simulink model "vfs_matlab"  (R2022a)
settings: Solver=FixedStepAuto  StartTime=0.0  StopTime=tend  FixedStep=0.02  RelTol=1e-3
undefined symbols (not defined in the file): alpha, center1, center2, center3, epsilon1, epsilon2, epsilon3, gd, Kc, psi0, pwo_init, scale1, scale2, scale3, switchingPoints, switchingWidth, T, v1, v2, v3, var_max
libraries: simlib_vpc_basic x23, simlib_vpc_coremath x14, simlib_vpc_gp x7
settings Model: Creator=marco  LastModifiedBy=marco
settings DebuggingCC: AlgebraicLoopMsg=none  ArtificialAlgebraicLoopMsg=none  UnconnectedInputMsg=warning  UnconnectedOutputMsg=warning  UnconnectedLineMsg=warning
settings RTWCC: DLArmComputeVersion=19.05

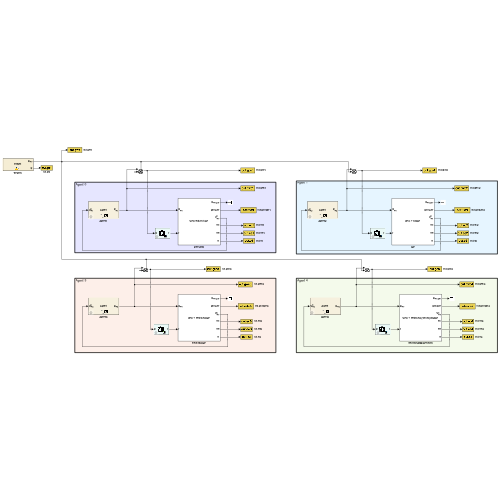
[thumbnail: Simulink's stored preview of the top-level diagram]
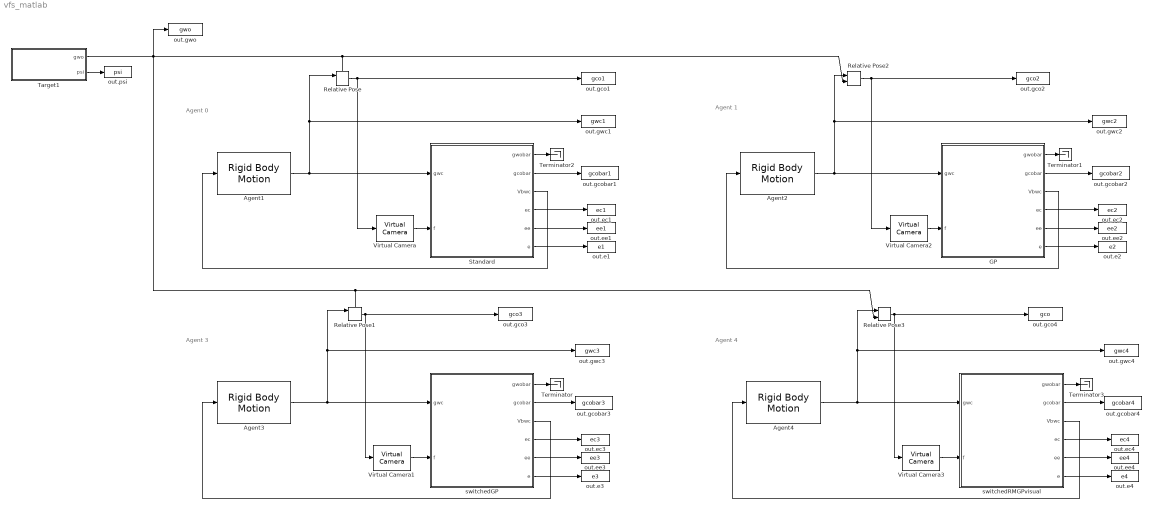
== system vfs_matlab ==
  note: Agent 3
  note: Agent 1
  note: Agent 0
  note: Agent 4
  Agent1 : simlib_vpc_basic/Rigid Body Motion  rbmtype=agent  agentnumber=1  projection=on  show_dg=off  g0=gwc_init
      settings: SourceProductName=VPC Library
  Agent2 : simlib_vpc_basic/Rigid Body Motion  rbmtype=agent  agentnumber=2  projection=on  show_dg=off  g0=gwc_init
      settings: SourceProductName=VPC Library
  Agent3 : simlib_vpc_basic/Rigid Body Motion  rbmtype=agent  agentnumber=3  projection=on  show_dg=off  g0=gwc_init
      settings: SourceProductName=VPC Library
  Agent4 : simlib_vpc_basic/Rigid Body Motion  rbmtype=agent  agentnumber=4  projection=on  show_dg=off  g0=gwc_init
      settings: SourceProductName=VPC Library
  GP : Subsystem
      mask Display:
      | disp('VPC + fullGP','texmode','on')
      | 
      | % Label ports
      | port_label('input',1,'g_{wc}','texmode','on')
      | port_label('input',2,'f','texmode','on')
      | port_label('output',1,'g_{wo,bar}','texmode','on')
      | port_label('output',2,'gco,bar','texmode','on')
      | port_label('output',3,'V^b_{wc}','texmode','on')
      | port_label('output',4,'ec','texmode','on')
      | port_label('output',5,'ee','texmode','on')
      | port_label('output',6,'e','texmode','on')
  Relative Pose{,1..3} (4 alike) : simlib_vpc_coremath/Relative Pose
      settings: SourceProductName=VPC Library
  Standard : Subsystem
      mask Display:
      | disp('VPC without GP','texmode','on')
      | 
      | % Label ports
      | port_label('input',1,'g_{wc}','texmode','on')
      | port_label('input',2,'f','texmode','on')
      | port_label('output',1,'g_{wo,bar}','texmode','on')
      | port_label('output',2,'gco,bar','texmode','on')
      | port_label('output',3,'V^b_{wc}','texmode','on')
      | port_label('output',4,'ec','texmode','on')
      | port_label('output',5,'ee','texmode','on')
      | port_label('output',6,'e','texmode','on')
  Target1 : Subsystem
      mask Display:
      | % Glitch in Matlab: If you define a line whose starting point and end point
      | % is equal, then the entire mask block is plotted in bold
      | plot([0,0],[0,0])
      | 
      | % Draw Box
      | plot([0,1,1,0,0],[0,0,1,1,0])
      | 
      | % Write label
      | disp('Target','texmode','on')
      | 
      | % Image
      | p=get_param(gcb,'Position');
      | size = min(p(3:4)-p(1:2));
      | blkscale = abs((p(3)-p(1)) / (p(4)-p(2)));
      | if abs((p(3)-p(1))) > abs((p(4)-p(2))) % block is horizontal
      |     scale = .5*[1/blkscale .6];
      | else % block is vertical
      |     scale = .5*[1 .6*blkscale];
      | end
      | pos = [1-scale(1) 0.1]/2;
      | image('ico_target.png',[pos scale],'off')
      | 
      | % Label ports
      | port_label('output',1,'g_{wo}','texmode','on')
      | port_label('output',2,'\psi','texmode','on')
  Terminator{,1..3} (4 alike) : Terminator
  Virtual Camera{,1..3} (4 alike) : simlib_vpc_basic/Virtual Camera  camtype=Pinhole  po=fp  lambda=lambda
      settings: SourceProductName=VPC Library
  out.e1 : ToWorkspace  VariableName=e1  SaveFormat=Structure With Time  SampleTime=-1
  out.e2 : ToWorkspace  VariableName=e2  SaveFormat=Structure With Time  SampleTime=-1
  out.e3 : ToWorkspace  VariableName=e3  SaveFormat=Structure With Time  SampleTime=-1
  out.e4 : ToWorkspace  VariableName=e4  SaveFormat=Structure With Time  SampleTime=-1
  out.ec1 : ToWorkspace  VariableName=ec1  SaveFormat=Structure With Time  SampleTime=-1
  out.ec2 : ToWorkspace  VariableName=ec2  SaveFormat=Structure With Time  SampleTime=-1
  out.ec3 : ToWorkspace  VariableName=ec3  SaveFormat=Structure With Time  SampleTime=-1
  out.ec4 : ToWorkspace  VariableName=ec4  SaveFormat=Structure With Time  SampleTime=-1
  out.ee1 : ToWorkspace  VariableName=ee1  SaveFormat=Structure With Time  SampleTime=-1
  out.ee2 : ToWorkspace  VariableName=ee2  SaveFormat=Structure With Time  SampleTime=-1
  out.ee3 : ToWorkspace  VariableName=ee3  SaveFormat=Structure With Time  SampleTime=-1
  out.ee4 : ToWorkspace  VariableName=ee4  SaveFormat=Structure With Time  SampleTime=-1
  out.gco1 : ToWorkspace  VariableName=gco1  SaveFormat=Structure With Time  SampleTime=-1
  out.gco2 : ToWorkspace  VariableName=gco2  SaveFormat=Structure With Time  SampleTime=-1
  out.gco3 : ToWorkspace  VariableName=gco3  SaveFormat=Structure With Time  SampleTime=-1
  out.gco4 : ToWorkspace  VariableName=gco  SaveFormat=Structure With Time  SampleTime=-1
  out.gcobar1 : ToWorkspace  VariableName=gcobar1  SaveFormat=Structure With Time  SampleTime=-1
  out.gcobar2 : ToWorkspace  VariableName=gcobar2  SaveFormat=Structure With Time  SampleTime=-1
  out.gcobar3 : ToWorkspace  VariableName=gcobar3  SaveFormat=Structure With Time  SampleTime=-1
  out.gcobar4 : ToWorkspace  VariableName=gcobar4  SaveFormat=Structure With Time  SampleTime=-1
  out.gwc1 : ToWorkspace  VariableName=gwc1  SaveFormat=Structure With Time  SampleTime=-1
  out.gwc2 : ToWorkspace  VariableName=gwc2  SaveFormat=Structure With Time  SampleTime=-1
  out.gwc3 : ToWorkspace  VariableName=gwc3  SaveFormat=Structure With Time  SampleTime=-1
  out.gwc4 : ToWorkspace  VariableName=gwc4  SaveFormat=Structure With Time  SampleTime=-1
  out.gwo : ToWorkspace  VariableName=gwo  SaveFormat=Structure With Time  SampleTime=-1
  out.psi : ToWorkspace  VariableName=psi  SaveFormat=Structure With Time  SampleTime=-1
  switchedGP : Subsystem
      mask Display:
      | disp('VPC + switchedGP','texmode','on')
      | 
      | % Label ports
      | port_label('input',1,'g_{wc}','texmode','on')
      | port_label('input',2,'f','texmode','on')
      | port_label('output',1,'g_{wo,bar}','texmode','on')
      | port_label('output',2,'gco,bar','texmode','on')
      | port_label('output',3,'V^b_{wc}','texmode','on')
      | port_label('output',4,'ec','texmode','on')
      | port_label('output',5,'ee','texmode','on')
      | port_label('output',6,'e','texmode','on')
  switchedRMGPvisual : Subsystem
      mask Display:
      | disp('VPC + switched (visual) RMGP','texmode','on')
      | 
      | % Label ports
      | port_label('input',1,'g_{wc}','texmode','on')
      | port_label('input',2,'f','texmode','on')
      | port_label('output',1,'g_{wo,bar}','texmode','on')
      | port_label('output',2,'gco,bar','texmode','on')
      | port_label('output',3,'V^b_{wc}','texmode','on')
      | port_label('output',4,'ec','texmode','on')
      | port_label('output',5,'ee','texmode','on')
      | port_label('output',6,'e','texmode','on')
  wires:
  Relative Pose2/1 -> Virtual Camera2/1, out.gco2/1
  Relative Pose/1 -> Virtual Camera/1, out.gco1/1
  GP/2(gcobar) -> out.gcobar2/1
  switchedGP/4(ec) -> out.ec3/1
  Relative Pose1/1 -> out.gco3/1, Virtual Camera1/1
  Agent3/1 -> switchedGP/1(gwc), out.gwc3/1, Relative Pose1/1
  Virtual Camera/1 -> Standard/2(f)
  switchedGP/2(gcobar) -> out.gcobar3/1
  Virtual Camera2/1 -> GP/2(f)
  switchedGP/5(ee) -> out.ee3/1
  GP/4(ec) -> out.ec2/1
  switchedGP/6(e) -> out.e3/1
  Virtual Camera1/1 -> switchedGP/2(f)
  Agent1/1 -> Standard/1(gwc), out.gwc1/1, Relative Pose/1
  Standard/6(e) -> out.e1/1
  Target1/1(gwo) -> Relative Pose2/2, Relative Pose/2, out.gwo/1, Relative Pose3/2, Relative Pose1/2
  Standard/4(ec) -> out.ec1/1
  Standard/5(ee) -> out.ee1/1
  Agent2/1 -> GP/1(gwc), out.gwc2/1, Relative Pose2/1
  Standard/2(gcobar) -> out.gcobar1/1
  GP/5(ee) -> out.ee2/1
  GP/6(e) -> out.e2/1
  Standard/3(Vbwc) -> Agent1/1
  switchedGP/3(Vbwc) -> Agent3/1
  GP/3(Vbwc) -> Agent2/1
  switchedGP/1(gwobar) -> Terminator/1
  GP/1(gwobar) -> Terminator1/1
  Standard/1(gwobar) -> Terminator2/1
  switchedRMGPvisual/4(ec) -> out.ec4/1
  switchedRMGPvisual/6(e) -> out.e4/1
  switchedRMGPvisual/5(ee) -> out.ee4/1
  Relative Pose3/1 -> out.gco4/1, Virtual Camera3/1
  switchedRMGPvisual/2(gcobar) -> out.gcobar4/1
  Agent4/1 -> switchedRMGPvisual/1(gwc), out.gwc4/1, Relative Pose3/1
  switchedRMGPvisual/3(Vbwc) -> Agent4/1
  Virtual Camera3/1 -> switchedRMGPvisual/2(f)
  switchedRMGPvisual/1(gwobar) -> Terminator3/1
  Target1/2(psi) -> out.psi/1

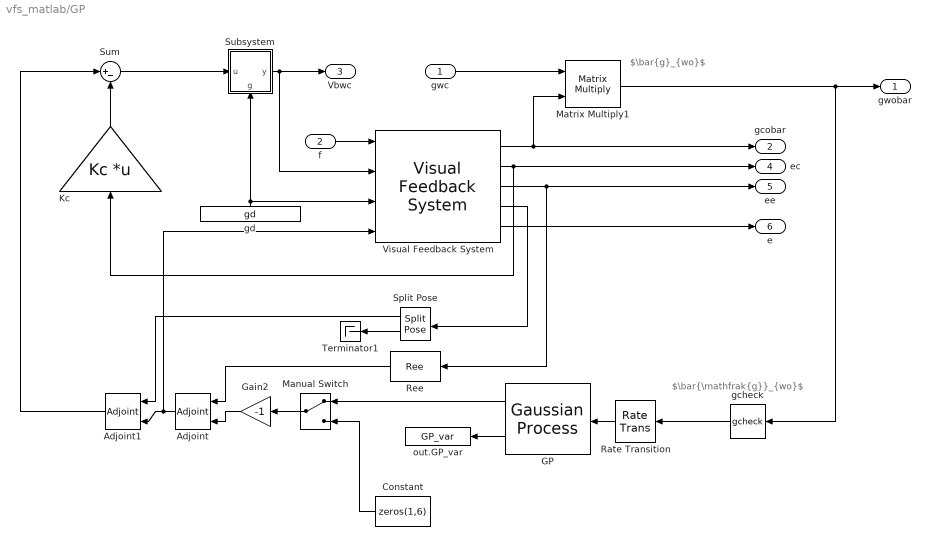
== system vfs_matlab/GP ==
  note: $\bar{g}_{wo}$
  note: $\bar{\mathfrak{g}}_{wo}$
  gwc : Inport
  f : Inport  Port=2
  Adjoint : simlib_vpc_basic/Adjoint  adjointtype=orientation
      settings: SourceProductName=VPC Library
  Adjoint1 : simlib_vpc_basic/Adjoint  adjointtype=orientation
      settings: SourceProductName=VPC Library
  Constant : Constant  Value=zeros(1,6)
  GP : simlib_vpc_gp/Gaussian Process  X=X_GP  Y=Y_GP  sn=sn_GP  kernel=Squared Exponential ARD  hyp=hyp_GP  show_mean=on  show_variance=on  inv_fallback=off
      settings: SourceProductName=VPC Library
  Gain2 : Gain  Gain=-1
  Kc : Gain  Gain=Kc  Multiplication=Matrix(K*u) (u vector)
  Manual Switch : ManualSwitch
  Matrix Multiply1 : Product  Multiplication=Matrix(*)
  Rate Transition : RateTransition
  Ree : simlib_vpc_coremath/Ree
      settings: SourceProductName=VPC Library
  Split Pose : simlib_vpc_coremath/Split Pose  show_R=on  show_p=on
      settings: SourceProductName=VPC Library
  Subsystem : Subsystem
      settings: PortSchema="{\"entries\":[{\"content\":{\"sides\":[{\"content\":{\"connectorIds\":[\"In1\"]},\"type\":\"ConnectorPlacement.EquallySpacedRectSide\",\"uuid\":\"72e68008-5c4a-43a9-a560-64c6a31a0c08\"},{\"content\":{\"connectorIds\":[\"Out1\"],\"side\":\"RIGHT\"},\"type\":\"ConnectorPlacement.EquallySpacedRectSide\",\"uuid\":\"da07f5ff-2b2c-4c55-a2f2-34e133777503\"},{\"content\":{\"connectorIds\":[],\"side\":\"TOP\"},\"type\":\"ConnectorPlacement.EquallySpacedRectSide\",\"uuid\":\"6d174428-4364-4e89-aba7-4e9864808ab5\"},{\"content\":{\"connectorIds\":[\"In2\"],\"side\":\"BOTTOM\"},\"type\":\"ConnectorPlacement.EquallySpacedRectSide\",\"uuid\":\"f9633104-9c11-4d21-90a7-e0f886d9e92d\"},{\"content\":{\"connectorIds\":[],\"side\":\"HIDDEN\"},\"type\":\"ConnectorPlacement.EquallySpacedRectSide\",\"uuid\":\"662f08ae-9279-4a4f-85ea-81d97ead27d9\"}]},\"type\":\"ConnectorPlacement.EquallySpacedConnector\",\"uuid\":\"f3cd156c-cccd-47c6-b81c-6113f78efd58\"}],\"packageUris\":[\"http://schema.mathworks.com/mf0/Connector/R2020b\"],\"version\":\"1.0\"}"
      mask Display:
      | % Glitch in Matlab: If you define a line whose starting point and end point
      | % is equal, then the entire mask block is plotted in bold
      | plot([0,0],[0,0])
      | 
      | % Draw box
      | indent = 0.3;
      | ang=[0:0.2:pi/2, pi/2];
      | plot([0,1-indent],[0,0])
      | xp=indent*sin(ang)+1-indent;
      | yp=indent-indent*cos(ang);
      | plot(xp,yp);
      | plot([1,1,indent],[indent,1,1])
      | xp=indent-indent*sin(ang);
      | yp=1-indent+indent*cos(ang);
      | plot(xp,yp);
      | plot([0,0],[1-indent,0])
      | 
      | % Write label & ports
      | disp('-Ad_{(g_d)}','texmode','on')
      | text(0.5,0.2,'\fontsize{7}g_d','texmode','on')
  Sum : Sum  Inputs=|+-
  Terminator1 : Terminator
  Visual Feedback System : simlib_vpc_basic/Visual Feedback System  gd_source=external  gd_value=[eye(4,3),ones(4,1)]  gcobar0=gco_init  Ke_source=internal  Ke=Ke  projection=on  camtype=Pinhole  fo=fp  lambda=lambda  show_Vbwo=off  show_ec=on  show_gce=on  show_ee=on  show_gee=off  show_e=on  show_nu=off  show_dgcobar=off  show_ue_aux=on
      settings: SourceProductName=VPC Library
  gcheck : simlib_vpc_coremath/gcheck
      settings: SourceProductName=VPC Library
  gd : Constant  Value=gd
  out.GP_var : ToWorkspace  VariableName=GP_var  SaveFormat=Structure With Time  SampleTime=-1
  gwobar : Outport
  gcobar : Outport  Port=2
  Vbwc : Outport  Port=3
  ec : Outport  Port=4
  ee : Outport  Port=5
  e : Outport  Port=6
  wires:
  f/1 -> Visual Feedback System/1
  Matrix Multiply1/1 -> gcheck/1, gwobar/1
  Subsystem/1(y) -> Vbwc/1, Visual Feedback System/2
  gwc/1 -> Matrix Multiply1/1
  Visual Feedback System/5 -> e/1
  Kc/1 -> Sum/2
  Visual Feedback System/2 -> ec/1, Kc/1
  Visual Feedback System/3 -> Ree/1, ee/1
  gd/1 -> Subsystem/2(g), Visual Feedback System/3
  Visual Feedback System/1 -> Matrix Multiply1/2, gcobar/1
  Split Pose/1 -> Adjoint1/2
  Rate Transition/1 -> GP/1
  Adjoint/1 -> Visual Feedback System/4, Adjoint1/1
  Ree/1 -> Adjoint/2
  Split Pose/2 -> Terminator1/1
  Gain2/1 -> Adjoint/1
  Manual Switch/1 -> Gain2/1
  Sum/1 -> Subsystem/1(u)
  Adjoint1/1 -> Sum/1
  Visual Feedback System/4 -> Split Pose/1
  GP/2 -> out.GP_var/1
  gcheck/1 -> Rate Transition/1
  GP/1 -> Manual Switch/1
  Constant/1 -> Manual Switch/2

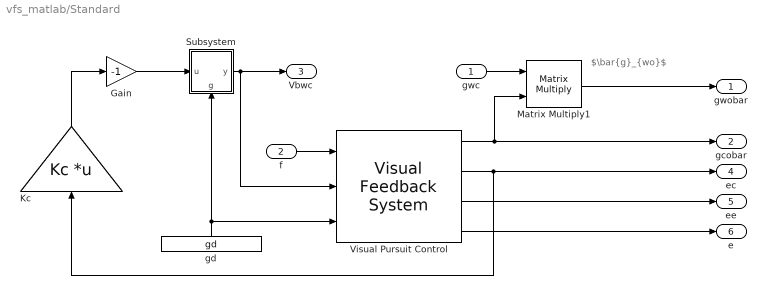
== system vfs_matlab/Standard ==
  note: $\bar{g}_{wo}$
  gwc : Inport
  f : Inport  Port=2
  Gain : Gain  Gain=-1
  Kc : Gain  Gain=Kc  Multiplication=Matrix(K*u) (u vector)
  Matrix Multiply1 : Product  Multiplication=Matrix(*)
  Subsystem : Subsystem
      settings: PortSchema="{\"entries\":[{\"content\":{\"sides\":[{\"content\":{\"connectorIds\":[\"In1\"]},\"type\":\"ConnectorPlacement.EquallySpacedRectSide\",\"uuid\":\"72e68008-5c4a-43a9-a560-64c6a31a0c08\"},{\"content\":{\"connectorIds\":[\"Out1\"],\"side\":\"RIGHT\"},\"type\":\"ConnectorPlacement.EquallySpacedRectSide\",\"uuid\":\"da07f5ff-2b2c-4c55-a2f2-34e133777503\"},{\"content\":{\"connectorIds\":[],\"side\":\"TOP\"},\"type\":\"ConnectorPlacement.EquallySpacedRectSide\",\"uuid\":\"6d174428-4364-4e89-aba7-4e9864808ab5\"},{\"content\":{\"connectorIds\":[\"In2\"],\"side\":\"BOTTOM\"},\"type\":\"ConnectorPlacement.EquallySpacedRectSide\",\"uuid\":\"f9633104-9c11-4d21-90a7-e0f886d9e92d\"},{\"content\":{\"connectorIds\":[],\"side\":\"HIDDEN\"},\"type\":\"ConnectorPlacement.EquallySpacedRectSide\",\"uuid\":\"662f08ae-9279-4a4f-85ea-81d97ead27d9\"}]},\"type\":\"ConnectorPlacement.EquallySpacedConnector\",\"uuid\":\"f3cd156c-cccd-47c6-b81c-6113f78efd58\"}],\"packageUris\":[\"http://schema.mathworks.com/mf0/Connector/R2020b\"],\"version\":\"1.0\"}"
      mask Display:
      | % Glitch in Matlab: If you define a line whose starting point and end point
      | % is equal, then the entire mask block is plotted in bold
      | plot([0,0],[0,0])
      | 
      | % Draw box
      | indent = 0.3;
      | ang=[0:0.2:pi/2, pi/2];
      | plot([0,1-indent],[0,0])
      | xp=indent*sin(ang)+1-indent;
      | yp=indent-indent*cos(ang);
      | plot(xp,yp);
      | plot([1,1,indent],[indent,1,1])
      | xp=indent-indent*sin(ang);
      | yp=1-indent+indent*cos(ang);
      | plot(xp,yp);
      | plot([0,0],[1-indent,0])
      | 
      | % Write label & ports
      | disp('-Ad_{(g_d)}','texmode','on')
      | text(0.5,0.2,'\fontsize{7}g_d','texmode','on')
  Visual Pursuit Control : simlib_vpc_basic/Visual Feedback System  gd_source=external  gd_value=[eye(4,3),ones(4,1)]  gcobar0=gco_init  Ke_source=internal  Ke=Ke  projection=on  camtype=Pinhole  fo=fp  lambda=lambda  show_Vbwo=off  show_ec=on  show_gce=off  show_ee=on  show_gee=off  show_e=on  show_nu=off  show_dgcobar=off  show_ue_aux=off
      settings: SourceProductName=VPC Library
  gd : Constant  Value=gd
  gwobar : Outport
  gcobar : Outport  Port=2
  Vbwc : Outport  Port=3
  ec : Outport  Port=4
  ee : Outport  Port=5
  e : Outport  Port=6
  wires:
  f/1 -> Visual Pursuit Control/1
  Matrix Multiply1/1 -> gwobar/1
  Subsystem/1(y) -> Vbwc/1, Visual Pursuit Control/2
  gwc/1 -> Matrix Multiply1/1
  Kc/1 -> Gain/1
  Visual Pursuit Control/4 -> e/1
  Gain/1 -> Subsystem/1(u)
  Visual Pursuit Control/2 -> ec/1, Kc/1
  Visual Pursuit Control/3 -> ee/1
  gd/1 -> Subsystem/2(g), Visual Pursuit Control/3
  Visual Pursuit Control/1 -> gcobar/1, Matrix Multiply1/2

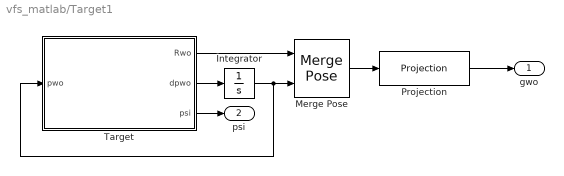
== system vfs_matlab/Target1 ==
  Integrator : Integrator  InitialCondition=pwo_init  ContinuousStateAttributes='pose'
  Merge Pose : simlib_vpc_coremath/Merge Pose
      settings: SourceProductName=VPC Library
  Projection : simlib_vpc_basic/Projection  projectiontype=averaging  inputtype=pose
      settings: SourceProductName=VPC Library
  Target : MATLAB Function  TreatAsAtomicUnit=on  SystemSampleTime=0.02
  gwo : Outport
  psi : Outport  Port=2
  wires:
  Target/1(Rwo) -> Merge Pose/1
  Target/2(dpwo) -> Integrator/1
  Integrator/1 -> Merge Pose/2, Target/1(pwo)
  Projection/1 -> gwo/1
  Merge Pose/1 -> Projection/1
  Target/3(psi) -> psi/1

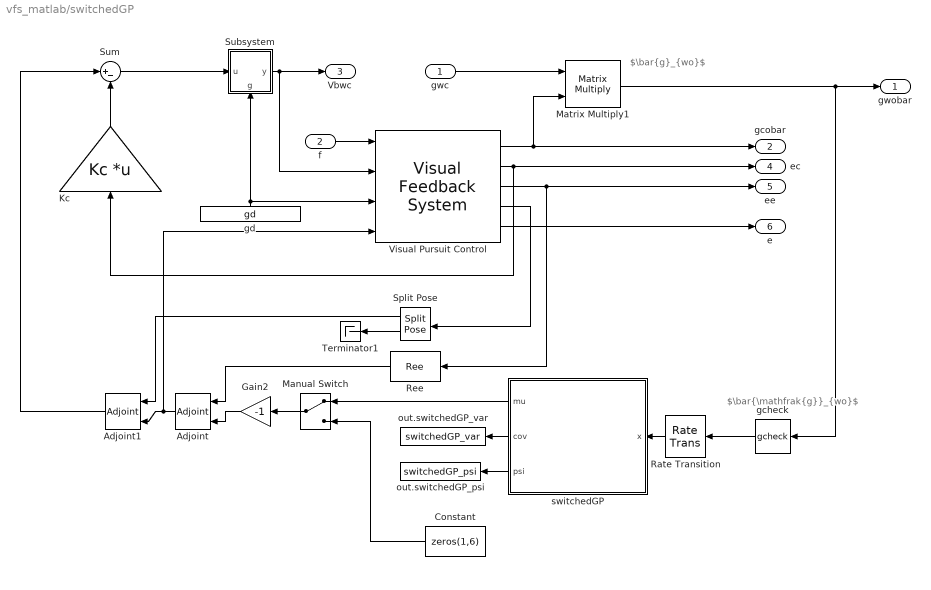
== system vfs_matlab/switchedGP ==
  note: $\bar{g}_{wo}$
  note: $\bar{\mathfrak{g}}_{wo}$
  gwc : Inport
  f : Inport  Port=2
  Adjoint : simlib_vpc_basic/Adjoint  adjointtype=orientation
      settings: SourceProductName=VPC Library
  Adjoint1 : simlib_vpc_basic/Adjoint  adjointtype=orientation
      settings: SourceProductName=VPC Library
  Constant : Constant  Value=zeros(1,6)
  Gain2 : Gain  Gain=-1
  Kc : Gain  Gain=Kc  Multiplication=Matrix(K*u) (u vector)
  Manual Switch : ManualSwitch
  Matrix Multiply1 : Product  Multiplication=Matrix(*)
  Rate Transition : RateTransition
  Ree : simlib_vpc_coremath/Ree
      settings: SourceProductName=VPC Library
  Split Pose : simlib_vpc_coremath/Split Pose  show_R=on  show_p=on
      settings: SourceProductName=VPC Library
  Subsystem : Subsystem
      settings: PortSchema="{\"entries\":[{\"content\":{\"sides\":[{\"content\":{\"connectorIds\":[\"In1\"]},\"type\":\"ConnectorPlacement.EquallySpacedRectSide\",\"uuid\":\"72e68008-5c4a-43a9-a560-64c6a31a0c08\"},{\"content\":{\"connectorIds\":[\"Out1\"],\"side\":\"RIGHT\"},\"type\":\"ConnectorPlacement.EquallySpacedRectSide\",\"uuid\":\"da07f5ff-2b2c-4c55-a2f2-34e133777503\"},{\"content\":{\"connectorIds\":[],\"side\":\"TOP\"},\"type\":\"ConnectorPlacement.EquallySpacedRectSide\",\"uuid\":\"6d174428-4364-4e89-aba7-4e9864808ab5\"},{\"content\":{\"connectorIds\":[\"In2\"],\"side\":\"BOTTOM\"},\"type\":\"ConnectorPlacement.EquallySpacedRectSide\",\"uuid\":\"f9633104-9c11-4d21-90a7-e0f886d9e92d\"},{\"content\":{\"connectorIds\":[],\"side\":\"HIDDEN\"},\"type\":\"ConnectorPlacement.EquallySpacedRectSide\",\"uuid\":\"662f08ae-9279-4a4f-85ea-81d97ead27d9\"}]},\"type\":\"ConnectorPlacement.EquallySpacedConnector\",\"uuid\":\"f3cd156c-cccd-47c6-b81c-6113f78efd58\"}],\"packageUris\":[\"http://schema.mathworks.com/mf0/Connector/R2020b\"],\"version\":\"1.0\"}"
      mask Display:
      | % Glitch in Matlab: If you define a line whose starting point and end point
      | % is equal, then the entire mask block is plotted in bold
      | plot([0,0],[0,0])
      | 
      | % Draw box
      | indent = 0.3;
      | ang=[0:0.2:pi/2, pi/2];
      | plot([0,1-indent],[0,0])
      | xp=indent*sin(ang)+1-indent;
      | yp=indent-indent*cos(ang);
      | plot(xp,yp);
      | plot([1,1,indent],[indent,1,1])
      | xp=indent-indent*sin(ang);
      | yp=1-indent+indent*cos(ang);
      | plot(xp,yp);
      | plot([0,0],[1-indent,0])
      | 
      | % Write label & ports
      | disp('-Ad_{(g_d)}','texmode','on')
      | text(0.5,0.2,'\fontsize{7}g_d','texmode','on')
  Sum : Sum  Inputs=|+-
  Terminator1 : Terminator
  Visual Pursuit Control : simlib_vpc_basic/Visual Feedback System  gd_source=external  gd_value=[eye(4,3),ones(4,1)]  gcobar0=gco_init  Ke_source=internal  Ke=Ke  projection=on  camtype=Pinhole  fo=fp  lambda=lambda  show_Vbwo=off  show_ec=on  show_gce=on  show_ee=on  show_gee=off  show_e=on  show_nu=off  show_dgcobar=off  show_ue_aux=on
      settings: SourceProductName=VPC Library
  gcheck : simlib_vpc_coremath/gcheck
      settings: SourceProductName=VPC Library
  gd : Constant  Value=gd
  out.switchedGP_psi : ToWorkspace  VariableName=switchedGP_psi  SaveFormat=Structure With Time  SampleTime=-1
  out.switchedGP_var : ToWorkspace  VariableName=switchedGP_var  SaveFormat=Structure With Time  SampleTime=-1
  switchedGP : Subsystem
      mask Display:
      | disp('Switched GP','texmode','on')
      | 
      | % Label ports
      | port_label('input',1,'x*','texmode','on')
      | port_label('output',1,'\mu','texmode','on')
      | port_label('output',2,'\Sigma','texmode','on')
      | port_label('output',3,'\psi_{est}','texmode','on')
  gwobar : Outport
  gcobar : Outport  Port=2
  Vbwc : Outport  Port=3
  ec : Outport  Port=4
  ee : Outport  Port=5
  e : Outport  Port=6
  wires:
  f/1 -> Visual Pursuit Control/1
  Matrix Multiply1/1 -> gcheck/1, gwobar/1
  Subsystem/1(y) -> Vbwc/1, Visual Pursuit Control/2
  gwc/1 -> Matrix Multiply1/1
  Visual Pursuit Control/5 -> e/1
  Kc/1 -> Sum/2
  Visual Pursuit Control/2 -> ec/1, Kc/1
  Visual Pursuit Control/3 -> Ree/1, ee/1
  gd/1 -> Subsystem/2(g), Visual Pursuit Control/3
  Visual Pursuit Control/1 -> Matrix Multiply1/2, gcobar/1
  Split Pose/1 -> Adjoint1/2
  Adjoint/1 -> Visual Pursuit Control/4, Adjoint1/1
  Ree/1 -> Adjoint/2
  Split Pose/2 -> Terminator1/1
  Gain2/1 -> Adjoint/1
  Sum/1 -> Subsystem/1(u)
  Adjoint1/1 -> Sum/1
  Visual Pursuit Control/4 -> Split Pose/1
  gcheck/1 -> Rate Transition/1
  switchedGP/3(psi) -> out.switchedGP_psi/1
  Rate Transition/1 -> switchedGP/1(x)
  switchedGP/2(cov) -> out.switchedGP_var/1
  switchedGP/1(mu) -> Manual Switch/1
  Manual Switch/1 -> Gain2/1
  Constant/1 -> Manual Switch/2

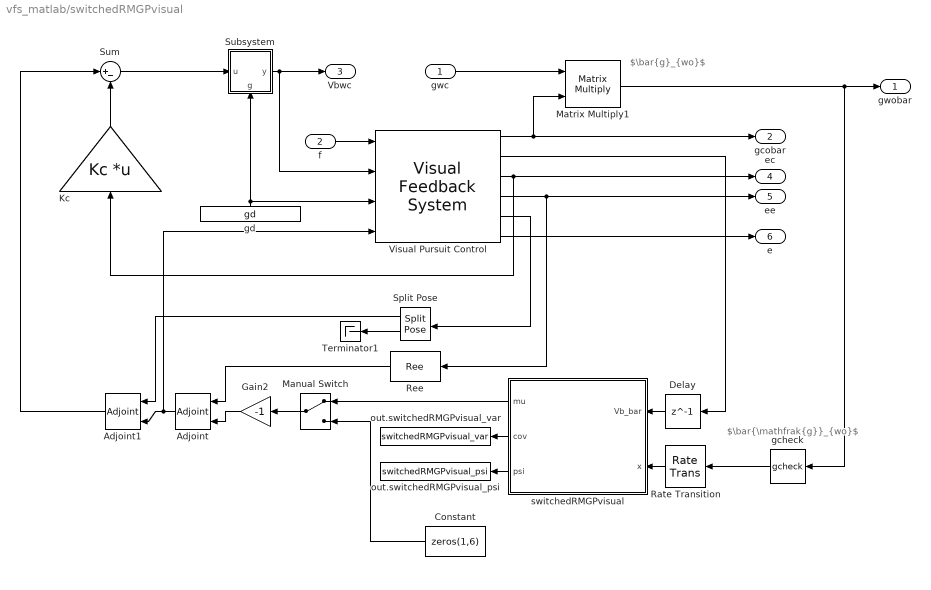
== system vfs_matlab/switchedRMGPvisual ==
  note: $\bar{g}_{wo}$
  note: $\bar{\mathfrak{g}}_{wo}$
  gwc : Inport
  f : Inport  Port=2
  Adjoint : simlib_vpc_basic/Adjoint  adjointtype=orientation
      settings: SourceProductName=VPC Library
  Adjoint1 : simlib_vpc_basic/Adjoint  adjointtype=orientation
      settings: SourceProductName=VPC Library
  Constant : Constant  Value=zeros(1,6)
  Delay : Delay  DelayLength=1
  Gain2 : Gain  Gain=-1
  Kc : Gain  Gain=Kc  Multiplication=Matrix(K*u) (u vector)
  Manual Switch : ManualSwitch
  Matrix Multiply1 : Product  Multiplication=Matrix(*)
  Rate Transition : RateTransition
  Ree : simlib_vpc_coremath/Ree
      settings: SourceProductName=VPC Library
  Split Pose : simlib_vpc_coremath/Split Pose  show_R=on  show_p=on
      settings: SourceProductName=VPC Library
  Subsystem : Subsystem
      settings: PortSchema="{\"entries\":[{\"content\":{\"sides\":[{\"content\":{\"connectorIds\":[\"In1\"]},\"type\":\"ConnectorPlacement.EquallySpacedRectSide\",\"uuid\":\"72e68008-5c4a-43a9-a560-64c6a31a0c08\"},{\"content\":{\"connectorIds\":[\"Out1\"],\"side\":\"RIGHT\"},\"type\":\"ConnectorPlacement.EquallySpacedRectSide\",\"uuid\":\"da07f5ff-2b2c-4c55-a2f2-34e133777503\"},{\"content\":{\"connectorIds\":[],\"side\":\"TOP\"},\"type\":\"ConnectorPlacement.EquallySpacedRectSide\",\"uuid\":\"6d174428-4364-4e89-aba7-4e9864808ab5\"},{\"content\":{\"connectorIds\":[\"In2\"],\"side\":\"BOTTOM\"},\"type\":\"ConnectorPlacement.EquallySpacedRectSide\",\"uuid\":\"f9633104-9c11-4d21-90a7-e0f886d9e92d\"},{\"content\":{\"connectorIds\":[],\"side\":\"HIDDEN\"},\"type\":\"ConnectorPlacement.EquallySpacedRectSide\",\"uuid\":\"662f08ae-9279-4a4f-85ea-81d97ead27d9\"}]},\"type\":\"ConnectorPlacement.EquallySpacedConnector\",\"uuid\":\"f3cd156c-cccd-47c6-b81c-6113f78efd58\"}],\"packageUris\":[\"http://schema.mathworks.com/mf0/Connector/R2020b\"],\"version\":\"1.0\"}"
      mask Display:
      | % Glitch in Matlab: If you define a line whose starting point and end point
      | % is equal, then the entire mask block is plotted in bold
      | plot([0,0],[0,0])
      | 
      | % Draw box
      | indent = 0.3;
      | ang=[0:0.2:pi/2, pi/2];
      | plot([0,1-indent],[0,0])
      | xp=indent*sin(ang)+1-indent;
      | yp=indent-indent*cos(ang);
      | plot(xp,yp);
      | plot([1,1,indent],[indent,1,1])
      | xp=indent-indent*sin(ang);
      | yp=1-indent+indent*cos(ang);
      | plot(xp,yp);
      | plot([0,0],[1-indent,0])
      | 
      | % Write label & ports
      | disp('-Ad_{(g_d)}','texmode','on')
      | text(0.5,0.2,'\fontsize{7}g_d','texmode','on')
  Sum : Sum  Inputs=|+-
  Terminator1 : Terminator
  Visual Pursuit Control : simlib_vpc_basic/Visual Feedback System  gd_source=external  gd_value=[eye(4,3),ones(4,1)]  gcobar0=gco_init  Ke_source=internal  Ke=Ke  projection=on  camtype=Pinhole  fo=fp  lambda=lambda  show_Vbwo=on  show_ec=on  show_gce=on  show_ee=on  show_gee=off  show_e=on  show_nu=off  show_dgcobar=off  show_ue_aux=on
      settings: SourceProductName=VPC Library
  gcheck : simlib_vpc_coremath/gcheck
      settings: SourceProductName=VPC Library
  gd : Constant  Value=gd
  out.switchedRMGPvisual_psi : ToWorkspace  VariableName=switchedRMGPvisual_psi  SaveFormat=Structure With Time  SampleTime=-1
  out.switchedRMGPvisual_var : ToWorkspace  VariableName=switchedRMGPvisual_var  SaveFormat=Structure With Time  SampleTime=-1
  switchedRMGPvisual : Subsystem
      mask Display:
      | disp('Switched GP','texmode','on')
      | 
      | % Label ports
      | port_label('input',1,'V^b_{est}','texmode','on')
      | port_label('input',2,'x*','texmode','on')
      | port_label('output',1,'\mu','texmode','on')
      | port_label('output',2,'\Sigma','texmode','on')
      | port_label('output',3,'\psi_{est}','texmode','on')
  gwobar : Outport
  gcobar : Outport  Port=2
  Vbwc : Outport  Port=3
  ec : Outport  Port=4
  ee : Outport  Port=5
  e : Outport  Port=6
  wires:
  f/1 -> Visual Pursuit Control/1
  Matrix Multiply1/1 -> gwobar/1, gcheck/1
  Subsystem/1(y) -> Vbwc/1, Visual Pursuit Control/2
  gwc/1 -> Matrix Multiply1/1
  Visual Pursuit Control/5 -> Split Pose/1
  Kc/1 -> Sum/2
  Visual Pursuit Control/3 -> ec/1, Kc/1
  Visual Pursuit Control/4 -> Ree/1, ee/1
  gd/1 -> Subsystem/2(g), Visual Pursuit Control/3
  Visual Pursuit Control/1 -> Matrix Multiply1/2, gcobar/1
  Split Pose/1 -> Adjoint1/2
  Adjoint/1 -> Visual Pursuit Control/4, Adjoint1/1
  Ree/1 -> Adjoint/2
  Split Pose/2 -> Terminator1/1
  Gain2/1 -> Adjoint/1
  Sum/1 -> Subsystem/1(u)
  Adjoint1/1 -> Sum/1
  Visual Pursuit Control/6 -> e/1
  gcheck/1 -> Rate Transition/1
  switchedRMGPvisual/3(psi) -> out.switchedRMGPvisual_psi/1
  Rate Transition/1 -> switchedRMGPvisual/2(x)
  switchedRMGPvisual/2(cov) -> out.switchedRMGPvisual_var/1
  switchedRMGPvisual/1(mu) -> Manual Switch/1
  Manual Switch/1 -> Gain2/1
  Constant/1 -> Manual Switch/2
  Delay/1 -> switchedRMGPvisual/1(Vb_bar)
  Visual Pursuit Control/2 -> Delay/1

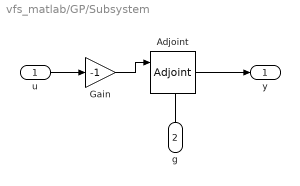
== system vfs_matlab/GP/Subsystem ==
  u : Inport
  g : Inport  Port=2
  Adjoint : simlib_vpc_basic/Adjoint  adjointtype=pose
      settings: SourceProductName=VPC Library
  Gain : Gain  Gain=-1
  y : Outport
  wires:
  Adjoint/1 -> y/1
  u/1 -> Gain/1
  g/1 -> Adjoint/2
  Gain/1 -> Adjoint/1

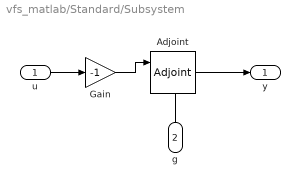
== system vfs_matlab/Standard/Subsystem ==
  u : Inport
  g : Inport  Port=2
  Adjoint : simlib_vpc_basic/Adjoint  adjointtype=pose
      settings: SourceProductName=VPC Library
  Gain : Gain  Gain=-1
  y : Outport
  wires:
  Adjoint/1 -> y/1
  u/1 -> Gain/1
  g/1 -> Adjoint/2
  Gain/1 -> Adjoint/1

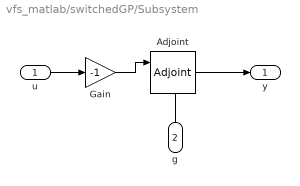
== system vfs_matlab/switchedGP/Subsystem ==
  u : Inport
  g : Inport  Port=2
  Adjoint : simlib_vpc_basic/Adjoint  adjointtype=pose
      settings: SourceProductName=VPC Library
  Gain : Gain  Gain=-1
  y : Outport
  wires:
  Adjoint/1 -> y/1
  u/1 -> Gain/1
  g/1 -> Adjoint/2
  Gain/1 -> Adjoint/1

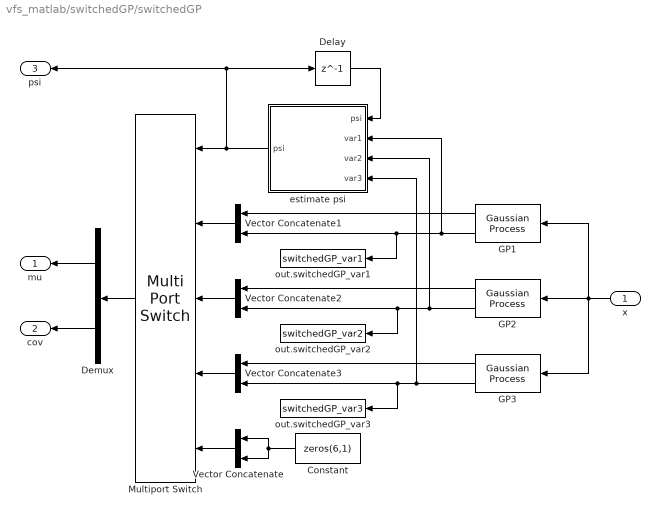
== system vfs_matlab/switchedGP/switchedGP ==
  x : Inport
  Constant : Constant  Value=zeros(6,1)
  Delay : Delay  DelayLength=1
  Demux : Demux  Outputs=2
  GP1 : simlib_vpc_gp/Gaussian Process  X=X_switchedGP1  Y=Y_switchedGP1  sn=sn_switchedGP1  kernel=Squared Exponential ARD  hyp=hyp_switchedGP1  show_mean=on  show_variance=on  inv_fallback=off
      settings: SourceProductName=VPC Library
  GP2 : simlib_vpc_gp/Gaussian Process  X=X_switchedGP2  Y=Y_switchedGP2  sn=sn_switchedGP2  kernel=Squared Exponential ARD  hyp=hyp_switchedGP2  show_mean=on  show_variance=on  inv_fallback=off
      settings: SourceProductName=VPC Library
  GP3 : simlib_vpc_gp/Gaussian Process  X=X_switchedGP3  Y=Y_switchedGP3  sn=sn_switchedGP3  kernel=Squared Exponential ARD  hyp=hyp_switchedGP3  show_mean=on  show_variance=on  inv_fallback=off
      settings: SourceProductName=VPC Library
  Multiport Switch : MultiPortSwitch  DataPortForDefault=Additional data port  SaturateOnIntegerOverflow=off  InputSameDT=off
  Vector Concatenate{,1..3} (4 alike) : Concatenate
  estimate psi : MATLAB Function  TreatAsAtomicUnit=on
  out.switchedGP_var1 : ToWorkspace  VariableName=switchedGP_var1  SaveFormat=Structure With Time  SampleTime=-1
  out.switchedGP_var2 : ToWorkspace  VariableName=switchedGP_var2  SaveFormat=Structure With Time  SampleTime=-1
  out.switchedGP_var3 : ToWorkspace  VariableName=switchedGP_var3  SaveFormat=Structure With Time  SampleTime=-1
  mu : Outport
  cov : Outport  Port=2
  psi : Outport  Port=3
  wires:
  Constant/1 -> Vector Concatenate/2, Vector Concatenate/1
  Vector Concatenate/1 -> Multiport Switch/5
  Vector Concatenate1/1 -> Multiport Switch/2
  Multiport Switch/1 -> Demux/1
  Vector Concatenate2/1 -> Multiport Switch/3
  GP2/1 -> Vector Concatenate2/1
  GP1/1 -> Vector Concatenate1/1
  GP2/2 -> out.switchedGP_var2/1, Vector Concatenate2/2, estimate psi/3(var2)
  GP1/2 -> estimate psi/2(var1), out.switchedGP_var1/1, Vector Concatenate1/2
  Demux/1 -> mu/1
  Demux/2 -> cov/1
  estimate psi/1(psi) -> Multiport Switch/1, psi/1, Delay/1
  Delay/1 -> estimate psi/1("psi ")
  Vector Concatenate3/1 -> Multiport Switch/4
  GP3/1 -> Vector Concatenate3/1
  x/1 -> GP1/1, GP3/1, GP2/1
  GP3/2 -> estimate psi/4(var3), out.switchedGP_var3/1, Vector Concatenate3/2

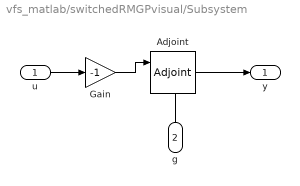
== system vfs_matlab/switchedRMGPvisual/Subsystem ==
  u : Inport
  g : Inport  Port=2
  Adjoint : simlib_vpc_basic/Adjoint  adjointtype=pose
      settings: SourceProductName=VPC Library
  Gain : Gain  Gain=-1
  y : Outport
  wires:
  Adjoint/1 -> y/1
  u/1 -> Gain/1
  g/1 -> Adjoint/2
  Gain/1 -> Adjoint/1

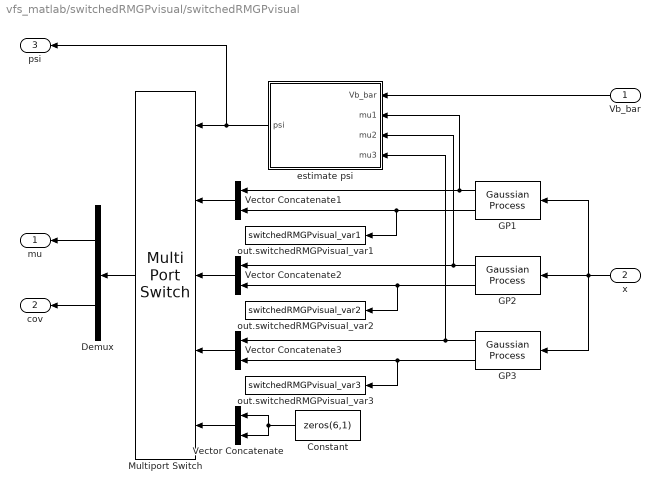
== system vfs_matlab/switchedRMGPvisual/switchedRMGPvisual ==
  Vb_bar : Inport
  x : Inport  Port=2
  Constant : Constant  Value=zeros(6,1)
  Demux : Demux  Outputs=2
  GP1 : simlib_vpc_gp/Gaussian Process  X=X_switchedRMGPvisual1  Y=Y_switchedRMGPvisual1  sn=sn_switchedRMGPvisual1  kernel=SE3  hyp=hyp_switchedRMGPvisual1  show_mean=on  show_variance=on  inv_fallback=off
      settings: SourceProductName=VPC Library
  GP2 : simlib_vpc_gp/Gaussian Process  X=X_switchedRMGPvisual2  Y=Y_switchedRMGPvisual2  sn=sn_switchedRMGPvisual2  kernel=SE3  hyp=hyp_switchedRMGPvisual2  show_mean=on  show_variance=on  inv_fallback=off
      settings: SourceProductName=VPC Library
  GP3 : simlib_vpc_gp/Gaussian Process  X=X_switchedRMGPvisual3  Y=Y_switchedRMGPvisual3  sn=sn_switchedRMGPvisual3  kernel=SE3  hyp=hyp_switchedRMGPvisual3  show_mean=on  show_variance=on  inv_fallback=off
      settings: SourceProductName=VPC Library
  Multiport Switch : MultiPortSwitch  DataPortForDefault=Additional data port  SaturateOnIntegerOverflow=off  InputSameDT=off
  Vector Concatenate{,1..3} (4 alike) : Concatenate
  estimate psi : MATLAB Function  TreatAsAtomicUnit=on
  out.switchedRMGPvisual_var1 : ToWorkspace  VariableName=switchedRMGPvisual_var1  SaveFormat=Structure With Time  SampleTime=-1
  out.switchedRMGPvisual_var2 : ToWorkspace  VariableName=switchedRMGPvisual_var2  SaveFormat=Structure With Time  SampleTime=-1
  out.switchedRMGPvisual_var3 : ToWorkspace  VariableName=switchedRMGPvisual_var3  SaveFormat=Structure With Time  SampleTime=-1
  mu : Outport
  cov : Outport  Port=2
  psi : Outport  Port=3
  wires:
  Constant/1 -> Vector Concatenate/1, Vector Concatenate/2
  Vector Concatenate/1 -> Multiport Switch/5
  Vector Concatenate1/1 -> Multiport Switch/2
  Multiport Switch/1 -> Demux/1
  Vector Concatenate2/1 -> Multiport Switch/3
  GP2/1 -> estimate psi/3(mu2), Vector Concatenate2/1
  GP1/1 -> estimate psi/2(mu1), Vector Concatenate1/1
  GP2/2 -> out.switchedRMGPvisual_var2/1, Vector Concatenate2/2
  GP1/2 -> out.switchedRMGPvisual_var1/1, Vector Concatenate1/2
  Demux/1 -> mu/1
  Demux/2 -> cov/1
  estimate psi/1(psi) -> psi/1, Multiport Switch/1
  Vb_bar/1 -> estimate psi/1(Vb_bar)
  Vector Concatenate3/1 -> Multiport Switch/4
  x/1 -> GP1/1, GP3/1, GP2/1
  GP3/2 -> out.switchedRMGPvisual_var3/1, Vector Concatenate3/2
  GP3/1 -> estimate psi/4(mu3), Vector Concatenate3/1

== matlab function vfs_matlab/switchedGP/switchedGP/estimate psi ==
  data: psi input; var1 input; psi output; var2 input; var3 input; var_max parameter; T parameter; alpha parameter
function psi = estim_psi(psi,var1,var2,var3,var_max,T,alpha)
%%ESTIM_PSI estimates the switching signal s(t)
%
% Editor:
%   OMAINSKA Marco - Doctoral Student, Cybernetics
%       <marcoomainska@g.ecc.u-tokyo.ac.jp>
% Review:
%   YAMAUCHI Junya - Assistant Professor
%       <junya_yamauchi@ipc.i.u-tokyo.ac.jp>
%
% Property of: Fujita-Yamauchi Lab, University of Tokyo, 2021
% e-mail: marcoomainska@g.ecc.u-tokyo.ac.jp
% Website: https://www.scl.ipc.i.u-tokyo.ac.jp
% February 2022
%
%------------- BEGIN CODE --------------

% calculate norms
var_norm = zeros(3,1);
% disp(var1);
var_norm(1) = norm(dot(alpha,sqrt(var1)),2)/var_max(1);
var_norm(2) = norm(dot(alpha,sqrt(var2)),2)/var_max(2);
var_norm(3) = norm(dot(alpha,sqrt(var3)),2)/var_max(3);

% estimate switching
if psi == 0 % init case: psi is zero
    [~,psi] = min(var_norm); % find the smallest ||var||/var_max
else
    [~,psi_new] = min(var_norm); % find the smallest ||var||/var_max
    if var_norm(psi) > var_norm(psi_new) + T
        psi = psi_new;
    end
end

% fail safe case
if isnan(psi)
    psi = 0;
end

%-------------- END CODE ---------------
end

== matlab function vfs_matlab/Target1/Target ==
  data: pwo input; epsilon1 parameter; epsilon2 parameter; v1 parameter; v2 parameter; scale1 parameter; Rwo output; dpwo output; scale2 parameter; center1 parameter; center2 parameter; psi output; switchingWidth parameter; switchingPoints parameter; psi0 parameter; scale3 parameter; v3 parameter; epsilon3 parameter; center3 parameter
function [Rwo, dpwo, psi] = target_trajectory(pwo, epsilon1, epsilon2, v1, v2, scale1, scale2, center1, center2, switchingWidth, switchingPoints, psi0, scale3, v3, epsilon3, center3) %#codegen
% Target Movement, Van-Der-Pol
%
% Editor:
%   OMAINSKA Marco - Doctoral Student, Cybernetics
%       <marcoomainska@g.ecc.u-tokyo.ac.jp>
% Review:
%   YAMAUCHI Junya - Assistant Professor
%       <junya_yamauchi@ipc.i.u-tokyo.ac.jp>
%
% Property of: Fujita-Yamauchi Lab, University of Tokyo, 2022
% e-mail: marcoomainska@g.ecc.u-tokyo.ac.jp
% Website: https://www.scl.ipc.i.u-tokyo.ac.jp
% March 2022
%
%------------- BEGIN CODE --------------

% config
% switchingWidth = 0.2;
% switchingPoints = [-2 0 0;
%                     2 0 0];

% init
persistent psi_ inside
if isempty(psi_) || isempty(inside)
    psi_ = psi0;
    inside = true;
end

% switch
insideNow = false;
for i = 1:size(switchingPoints,1)
    point = switchingPoints(i,:);
    p_dist = pwo(:) - point(:);
    if dot(p_dist,p_dist) <= switchingWidth*switchingWidth
        insideNow = true;
    end
end
if ~inside && insideNow
    psi_ = psi_+1;
end
if psi_ > 3
    psi_ = 1;
end
psi = psi_;
inside = insideNow;


% Get velocity
switch psi_
    case 1 % VF1
        Vb = vanderpol(pwo,v1,epsilon1,center1,scale1);
    case 2 % VF2
        Vb = vanderpol(pwo,v2,epsilon2,center2,scale2);
    case 3 % VF3
        Vb = vanderpol(pwo,v3,epsilon3,center3,scale3);
    otherwise % VF1
        Vb = vanderpol(pwo,v1,epsilon1,center1,scale1);
end
dpwo = Vb(1:3);

% set heading angle
angle = rad2deg(atan2(dpwo(2),dpwo(1)) - pi/2);
Rwo = rotz(angle);

%------------- END CODE --------------
end

== matlab function vfs_matlab/switchedRMGPvisual/switchedRMGPvisual/estimate psi ==
  data: Vb_bar input; mu1 input; psi output; mu2 input; mu3 input
function psi = estim_psi(Vb_bar,mu1,mu2,mu3)
%%ESTIM_PSI estimates the switching signal s(t)
%
% Editor:
%   OMAINSKA Marco - Doctoral Student, Cybernetics
%       <marcoomainska@g.ecc.u-tokyo.ac.jp>
% Review:
%   YAMAUCHI Junya - Assistant Professor
%       <junya_yamauchi@ipc.i.u-tokyo.ac.jp>
%
% Property of: Fujita-Yamauchi Lab, University of Tokyo, 2021
% e-mail: marcoomainska@g.ecc.u-tokyo.ac.jp
% Website: https://www.scl.ipc.i.u-tokyo.ac.jp
% February 2022
%
%------------- BEGIN CODE --------------

Vbee_vec = zeros(1,3);
Vbee_vec(1) = norm(Vb_bar-mu1,2);
Vbee_vec(2) = norm(Vb_bar-mu2,2);
Vbee_vec(3) = norm(Vb_bar-mu3,2);

[~,psi] = min(Vbee_vec);

%-------------- END CODE ---------------
end
